simulink model "OpenLoopTest"  (R2022b)
settings: Solver=VariableStepAuto  StartTime=0.0  StopTime=30  RelTol=1e-3
values from neighbouring files (symbols this model uses):
  B = (1/438)*(60/(2*pi))*1e-3    (= 2.18020469989e-05)    [GeneralParameters_PID_LQR.m]    (also in Rw_parameters.m = 1; System3x3.m = [5e-6 40e-6 1e-6])
  Iw = [1 0 0 ; 0 1 0; 0 0 1]    [Rw_parameters.m]
  Ke = (1/1120)*(60/(2*pi))    (= 0.00852615766564)    [GeneralParameters_PID_LQR.m]    (also in Rw_parameters.m = 1)
  Kt = 8.55e-3    (= 0.00855)    [GeneralParameters_PID_LQR.m]    (also in Rw_parameters.m = 1)
  La = 0.222e-3    (= 0.000222)    [GeneralParameters_PID_LQR.m]    (also in Rw_parameters.m = 10)
  Ra = 3.36    [GeneralParameters_PID_LQR.m]    (also in Rw_parameters.m = 100)
libraries: simulink_extras x3
settings Model: Creator=Personal  LastModifiedBy=Personal

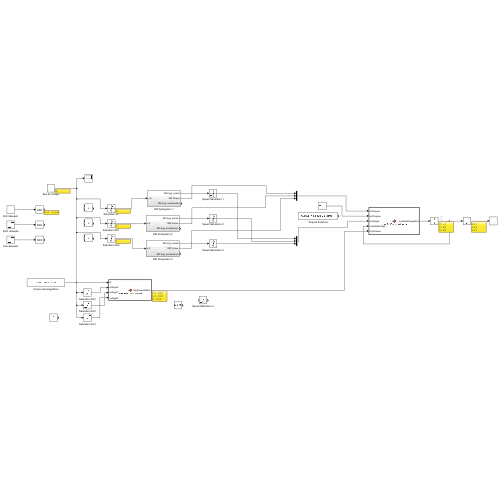
[thumbnail: Simulink's stored preview of the top-level diagram]
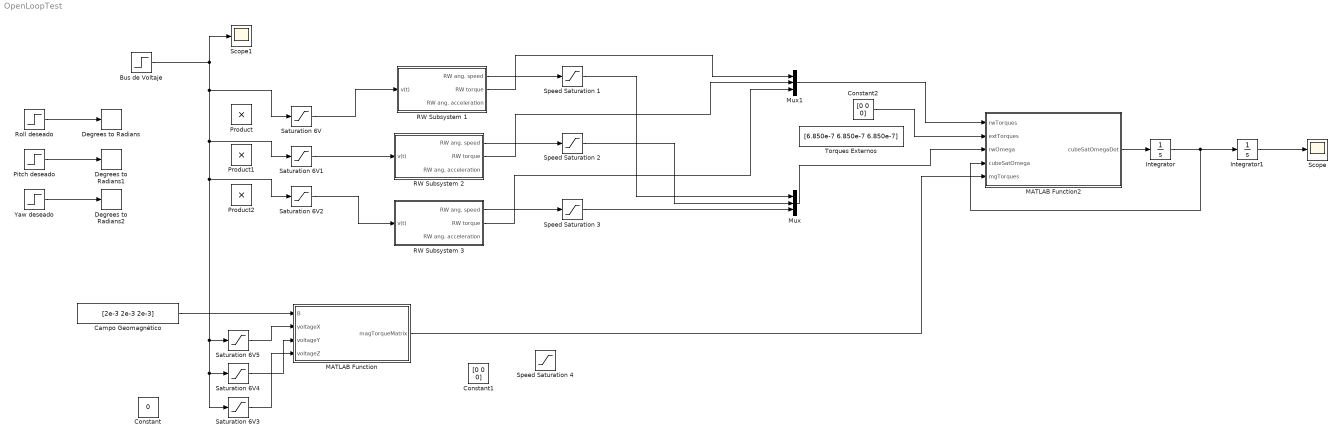
== system OpenLoopTest ==
  Bus de Voltaje : Step  Time=3  After=6  SampleTime=0
  Campo Geomagnético : Constant  Value=[2e-3 2e-3 2e-3]
  Constant : Constant  Value=0
  Constant1 : Constant  Value=[0 0 0]
  Constant2 : Constant  Value=[0 0 0]
  Degrees to Radians : simulink_extras/Transformations/Degrees to Radians
  Degrees to Radians1 : simulink_extras/Transformations/Degrees to Radians
  Degrees to Radians2 : simulink_extras/Transformations/Degrees to Radians
  Integrator : Integrator  InitialCondition=[0 0 0]
  Integrator1 : Integrator  InitialCondition=[0 0 0]
  MATLAB Function : MATLAB Function  TreatAsAtomicUnit=on
  MATLAB Function2 : MATLAB Function  TreatAsAtomicUnit=on
  Mux : Mux  Inputs=3
  Mux1 : Mux  Inputs=3
  Pitch deseado : Step  Time=2  After=0  SampleTime=0
  Product : Product
  Product1 : Product
  Product2 : Product
  RW Subsystem 1 : Subsystem
  RW Subsystem 2 : Subsystem
  RW Subsystem 3 : Subsystem
  Roll deseado : Step  Time=2  After=90  SampleTime=0
  Saturation 6V : Saturate  UpperLimit=6  LowerLimit=0
  Saturation 6V1 : Saturate  UpperLimit=2  LowerLimit=-6
  Saturation 6V2 : Saturate  UpperLimit=1  LowerLimit=-6
  Saturation 6V3 : Saturate  UpperLimit=3  LowerLimit=-6
  Saturation 6V4 : Saturate  UpperLimit=2  LowerLimit=-6
  Saturation 6V5 : Saturate  UpperLimit=6  LowerLimit=-6
  Scope : Scope
  Scope1 : Scope
  Speed Saturation {1..4} (4 alike) : Saturate  UpperLimit=8000  LowerLimit=0
  Torques Externos : Constant  Value=[6.850e-7 6.850e-7 6.850e-7]
  Yaw deseado : Step  Time=2  After=180  SampleTime=0
  wires:
  Roll deseado/1 -> Degrees to Radians/1
  Yaw deseado/1 -> Degrees to Radians2/1
  Pitch deseado/1 -> Degrees to Radians1/1
  Bus de Voltaje/1 -> Scope1/1, Saturation 6V/1, Saturation 6V1/1, Saturation 6V3/1, Saturation 6V4/1, Saturation 6V5/1, Saturation 6V2/1
  Saturation 6V/1 -> RW Subsystem 1/1(v(t))
  Saturation 6V1/1 -> RW Subsystem 2/1(v(t))
  Saturation 6V2/1 -> RW Subsystem 3/1(v(t))
  RW Subsystem 1/1(RW ang. speed) -> Speed Saturation 1/1
  RW Subsystem 2/1(RW ang. speed) -> Speed Saturation 2/1
  RW Subsystem 3/1(RW ang. speed) -> Speed Saturation 3/1
  RW Subsystem 1/2(RW torque) -> Mux1/1
  RW Subsystem 2/2(RW torque) -> Mux1/2
  RW Subsystem 3/2(RW torque) -> Mux1/3
  Speed Saturation 1/1 -> Mux/1
  Speed Saturation 2/1 -> Mux/2
  Speed Saturation 3/1 -> Mux/3
  MATLAB Function2/1(cubeSatOmegaDot) -> Integrator/1
  Integrator/1 -> Integrator1/1, MATLAB Function2/4(cubeSatOmega)
  Integrator1/1 -> Scope/1
  Mux/1 -> MATLAB Function2/3(rwOmega)
  Mux1/1 -> MATLAB Function2/1(rwTorques)
  Constant2/1 -> MATLAB Function2/2(extTorques)
  MATLAB Function/1(magTorqueMatrix) -> MATLAB Function2/5(mgTorques)
  Campo Geomagnético/1 -> MATLAB Function/1(B)
  Saturation 6V5/1 -> MATLAB Function/2(voltageX)
  Saturation 6V4/1 -> MATLAB Function/3(voltageY)
  Saturation 6V3/1 -> MATLAB Function/4(voltageZ)

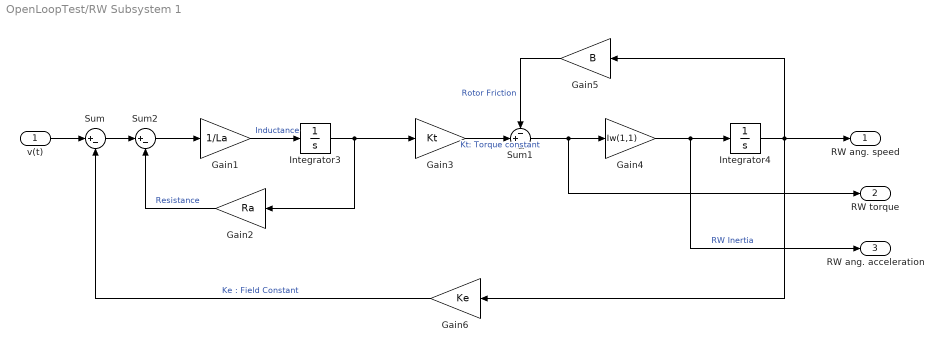
== system OpenLoopTest/RW Subsystem 1 ==
  v(t) : Inport
  Gain1 : Gain  Gain=1/La
  Gain2 : Gain  Gain=Ra
  Gain3 : Gain  Gain=Kt
  Gain4 : Gain  Gain=Iw(1,1)
  Gain5 : Gain  Gain=B
  Gain6 : Gain  Gain=Ke
  Integrator3 : Integrator
  Integrator4 : Integrator
  Sum : Sum  Inputs=|+-
  Sum1 : Sum  Inputs=-+|
  Sum2 : Sum  Inputs=|+-
  RW ang. speed : Outport  VectorParamsAs1DForOutWhenUnconnected=off
  RW torque : Outport  Port=2  VectorParamsAs1DForOutWhenUnconnected=off
  RW ang. acceleration : Outport  Port=3  VectorParamsAs1DForOutWhenUnconnected=off
  wires:
  Gain2/1 -> Sum2/2  "Resistance"
  Integrator3/1 -> Gain2/1, Gain3/1
  Gain6/1 -> Sum/2  "Ke : Field Constant"
  Gain5/1 -> Sum1/1  "Rotor Friction"
  v(t)/1 -> Sum/1
  Sum2/1 -> Gain1/1
  Sum1/1 -> Gain4/1, RW torque/1
  Integrator4/1 -> Gain5/1, Gain6/1, RW ang. speed/1
  Gain4/1 -> Integrator4/1, RW ang. acceleration/1  "RW Inertia"
  Gain1/1 -> Integrator3/1  "Inductance"
  Gain3/1 -> Sum1/2  "Kt: Torque constant"
  Sum/1 -> Sum2/1

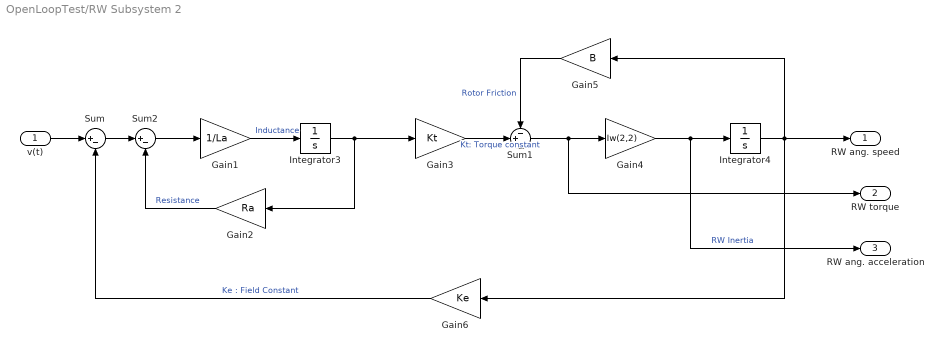
== system OpenLoopTest/RW Subsystem 2 ==
  v(t) : Inport
  Gain1 : Gain  Gain=1/La
  Gain2 : Gain  Gain=Ra
  Gain3 : Gain  Gain=Kt
  Gain4 : Gain  Gain=Iw(2,2)
  Gain5 : Gain  Gain=B
  Gain6 : Gain  Gain=Ke
  Integrator3 : Integrator
  Integrator4 : Integrator
  Sum : Sum  Inputs=|+-
  Sum1 : Sum  Inputs=-+|
  Sum2 : Sum  Inputs=|+-
  RW ang. speed : Outport  VectorParamsAs1DForOutWhenUnconnected=off
  RW torque : Outport  Port=2  VectorParamsAs1DForOutWhenUnconnected=off
  RW ang. acceleration : Outport  Port=3  VectorParamsAs1DForOutWhenUnconnected=off
  wires:
  Sum/1 -> Sum2/1
  Gain3/1 -> Sum1/2  "Kt: Torque constant"
  Gain1/1 -> Integrator3/1  "Inductance"
  Gain4/1 -> RW ang. acceleration/1, Integrator4/1  "RW Inertia"
  Integrator4/1 -> RW ang. speed/1, Gain6/1, Gain5/1
  Sum1/1 -> RW torque/1, Gain4/1
  Sum2/1 -> Gain1/1
  v(t)/1 -> Sum/1
  Gain5/1 -> Sum1/1  "Rotor Friction"
  Gain6/1 -> Sum/2  "Ke : Field Constant"
  Integrator3/1 -> Gain3/1, Gain2/1
  Gain2/1 -> Sum2/2  "Resistance"

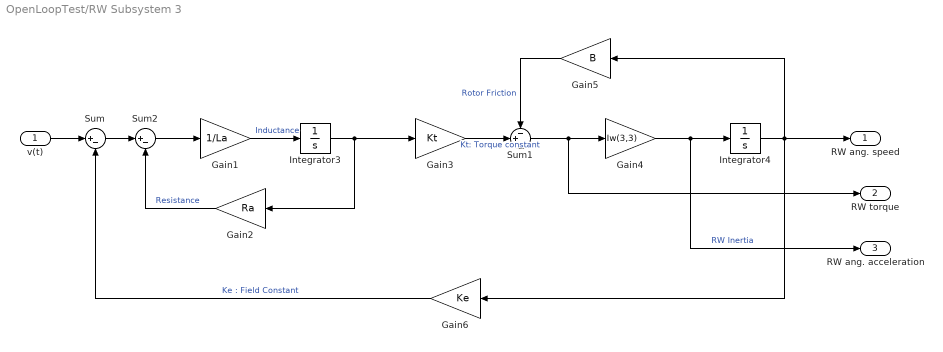
== system OpenLoopTest/RW Subsystem 3 ==
  v(t) : Inport
  Gain1 : Gain  Gain=1/La
  Gain2 : Gain  Gain=Ra
  Gain3 : Gain  Gain=Kt
  Gain4 : Gain  Gain=Iw(3,3)
  Gain5 : Gain  Gain=B
  Gain6 : Gain  Gain=Ke
  Integrator3 : Integrator
  Integrator4 : Integrator
  Sum : Sum  Inputs=|+-
  Sum1 : Sum  Inputs=-+|
  Sum2 : Sum  Inputs=|+-
  RW ang. speed : Outport  VectorParamsAs1DForOutWhenUnconnected=off
  RW torque : Outport  Port=2  VectorParamsAs1DForOutWhenUnconnected=off
  RW ang. acceleration : Outport  Port=3  VectorParamsAs1DForOutWhenUnconnected=off
  wires:
  Gain2/1 -> Sum2/2  "Resistance"
  Integrator3/1 -> Gain2/1, Gain3/1
  Gain6/1 -> Sum/2  "Ke : Field Constant"
  Gain5/1 -> Sum1/1  "Rotor Friction"
  v(t)/1 -> Sum/1
  Sum2/1 -> Gain1/1
  Sum1/1 -> Gain4/1, RW torque/1
  Integrator4/1 -> Gain5/1, Gain6/1, RW ang. speed/1
  Gain4/1 -> Integrator4/1, RW ang. acceleration/1  "RW Inertia"
  Gain1/1 -> Integrator3/1  "Inductance"
  Gain3/1 -> Sum1/2  "Kt: Torque constant"
  Sum/1 -> Sum2/1

== matlab function OpenLoopTest/MATLAB Function ==
  data: B input; magTorqueMatrix output; voltageX input; voltageY input; voltageZ input
function magTorqueMatrix = magTorqueFunction(B,voltageX,voltageY,voltageZ)

n=100;
R = 1000;
ix = voltageX/R;
iy = voltageY/R;
iz = voltageZ/R;

A =10;



magTorqueMatrix_X = cross(n*ix*A*[1 0 0],B);
magTorqueMatrix_Y = cross(n*iy*A*[0 1 0],B);
magTorqueMatrix_Z = cross(n*iz*A*[0 0 1],B);

magTorqueMatrix = magTorqueMatrix_X+magTorqueMatrix_Y+magTorqueMatrix_Z;

== matlab function OpenLoopTest/MATLAB Function2 ==
  data: rwTorques input; cubeSatOmegaDot output; extTorques input; rwOmega input; cubeSatOmega input; mgTorques input
function cubeSatOmegaDot = cubeSatDynamicModel(rwTorques,extTorques,rwOmega,cubeSatOmega,mgTorques)

% Inercia EyasSat [kg m2]
I =(4*0.3^2/6)*[1 0 0 ; 0 1 0; 0 0 1];

%Momentos de inercia EyasSat
Ixx = I(1,1);
Iyy = I(2,2);
Izz = I(3,3);

% Inercia EyasSat [kg m2]
Iw = 3e-6*[1 0 0 ; 0 1 0; 0 0 1]; %kg m2

%Momento angular RW
hw = Iw*rwOmega;

%Velocidades angulares EyasSat
wx = cubeSatOmega(1);
wy = cubeSatOmega(2);
wz = cubeSatOmega(3);

%Torques externos
Tx = extTorques(1);
Ty = extTorques(2);
Tz = extTorques(3);

%Torques de control RW
Tc_x = rwTorques(1);
Tc_y = rwTorques(2);
Tc_z = rwTorques(3);

%Torques de control RW
Tmg_x = mgTorques(1);
Tmg_y = mgTorques(2);
Tmg_z = mgTorques(3);

hx = hw(1);
hy = hw(2);
hz = hw(3);



omegaDotX = (Tx+Tc_x+Tmg_x+wy*wz*(Iyy-Izz)-hz*wy+hy*wz)/Ixx;
omegaDotY = (Ty+Tc_y+Tmg_y+wx*wz*(Izz-Ixx)-hx*wz+hz*wx)/Iyy;
omegaDotZ = (Tz+Tc_z+Tmg_z+wx*wy*(Ixx-Iyy)-hy*wx+hx*wy)/Izz;

cubeSatOmegaDot = [omegaDotX omegaDotY omegaDotZ];
